simulink model "test_11111"  (R2015a)
settings: Solver=ode45  StartTime=0.0  StopTime=311700  RelTol=1e-3
InitFcn:
  | %% DSPBuilder Start
  | alt_dspbuilder_update_model(bdroot)
  | %% DSPBuilder End
libraries: allblocks_alteradspbuilder2 x104
(part 1 of 2)
settings Model: Creator=ASUS  LastModifiedBy=ASUS

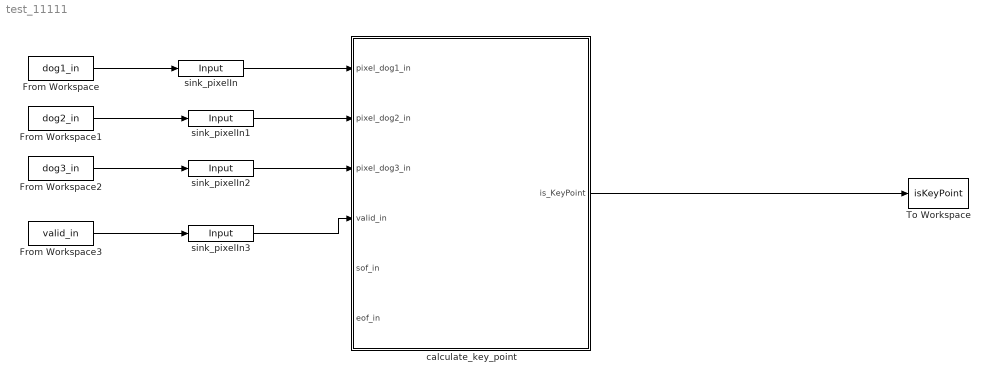
== system test_11111 ==
  From Workspace : FromWorkspace  VariableName=dog1_in  SampleTime=0
  From Workspace1 : FromWorkspace  VariableName=dog2_in  SampleTime=0
  From Workspace2 : FromWorkspace  VariableName=dog3_in  SampleTime=0
  From Workspace3 : FromWorkspace  VariableName=valid_in  SampleTime=0
  To Workspace : ToWorkspace  VariableName=isKeyPoint  SaveFormat=Timeseries  SampleTime=-1
  calculate_key_point : Subsystem
  sink_pixelIn : allblocks_alteradspbuilder2/Input  iofile=C:\Users\ASUS\Desktop\sift_fpga_final\Gaussian filter 5x5\tb_test_11111\test%5F11111_sink%5FpixelIn.salt  BusType=Signed Fractional  bwl=9  bwr=16  SpecifyClock=off  PORTTYPE=Input  externalType=Inferred  allowFloatingPointOverride=on  logOutputs=off
  sink_pixelIn1 : allblocks_alteradspbuilder2/Input  iofile=C:\Users\ASUS\Desktop\sift_fpga_final\Gaussian filter 5x5\tb_test_11111\test%5F11111_sink%5FpixelIn1.salt  BusType=Signed Fractional  bwl=9  bwr=16  SpecifyClock=off  PORTTYPE=Input  externalType=Inferred  allowFloatingPointOverride=on  logOutputs=off
  sink_pixelIn2 : allblocks_alteradspbuilder2/Input  iofile=C:\Users\ASUS\Desktop\sift_fpga_final\Gaussian filter 5x5\tb_test_11111\test%5F11111_sink%5FpixelIn2.salt  BusType=Signed Fractional  bwl=9  bwr=16  SpecifyClock=off  PORTTYPE=Input  externalType=Inferred  allowFloatingPointOverride=on  logOutputs=off
  sink_pixelIn3 : allblocks_alteradspbuilder2/Input  iofile=C:\Users\ASUS\Desktop\sift_fpga_final\Gaussian filter 5x5\tb_test_11111\test%5F11111_sink%5FpixelIn3.salt  BusType=Single Bit  bwl=8  bwr=0  SpecifyClock=off  PORTTYPE=Input  externalType=Inferred  allowFloatingPointOverride=on  logOutputs=off
  wires:
  From Workspace/1 -> sink_pixelIn/1
  From Workspace1/1 -> sink_pixelIn1/1
  From Workspace2/1 -> sink_pixelIn2/1
  From Workspace3/1 -> sink_pixelIn3/1
  calculate_key_point/1(is_KeyPoint) -> To Workspace/1
  sink_pixelIn/1 -> calculate_key_point/1(pixel_dog1_in)
  sink_pixelIn1/1 -> calculate_key_point/2(pixel_dog2_in)
  sink_pixelIn2/1 -> calculate_key_point/3(pixel_dog3_in)
  sink_pixelIn3/1 -> calculate_key_point/4(valid_in)

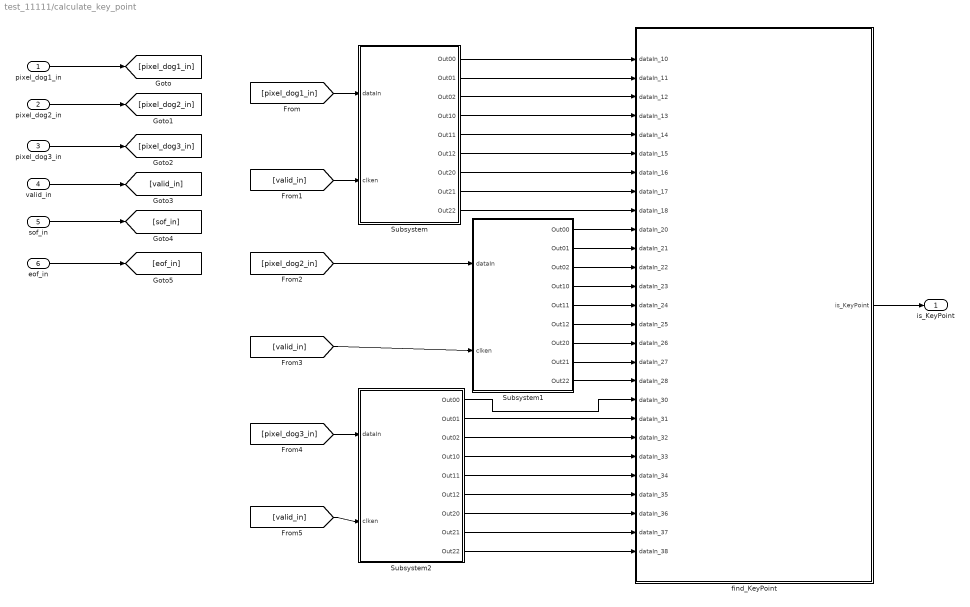
== system test_11111/calculate_key_point ==
  pixel_dog1_in : Inport
  pixel_dog2_in : Inport  Port=2
  pixel_dog3_in : Inport  Port=3
  valid_in : Inport  Port=4
  sof_in : Inport  Port=5
  eof_in : Inport  Port=6
  Subsystem : Subsystem
  Subsystem1 : Subsystem
  Subsystem2 : Subsystem
  find_KeyPoint : Subsystem
  is_KeyPoint : Outport
  wires:
  Subsystem/3(Out02) -> find_KeyPoint/3(dataIn_12)
  Subsystem/6(Out12) -> find_KeyPoint/6(dataIn_15)
  Subsystem/4(Out10) -> find_KeyPoint/4(dataIn_13)
  Subsystem/5(Out11) -> find_KeyPoint/5(dataIn_14)
  Subsystem1/2(Out01) -> find_KeyPoint/11(dataIn_21)
  Subsystem1/3(Out02) -> find_KeyPoint/12(dataIn_22)
  Subsystem1/4(Out10) -> find_KeyPoint/13(dataIn_23)
  Subsystem/2(Out01) -> find_KeyPoint/2(dataIn_11)
  Subsystem2/8(Out21) -> find_KeyPoint/26(dataIn_37)
  Subsystem/8(Out21) -> find_KeyPoint/8(dataIn_17)
  Subsystem/1(Out00) -> find_KeyPoint/1(dataIn_10)
  Subsystem/7(Out20) -> find_KeyPoint/7(dataIn_16)
  Subsystem/9(Out22) -> find_KeyPoint/9(dataIn_18)
  Subsystem1/1(Out00) -> find_KeyPoint/10(dataIn_20)
  find_KeyPoint/1(is_KeyPoint) -> is_KeyPoint/1
  Subsystem2/7(Out20) -> find_KeyPoint/25(dataIn_36)
  [pixel_dog2_in] -> Subsystem1/1(dataIn)
  [pixel_dog1_in] -> Subsystem/1(dataIn)
  eof_in/1 -> [eof_in]
  [valid_in] -> Subsystem2/2(clken)
  valid_in/1 -> [valid_in]
  [valid_in] -> Subsystem1/2(clken)
  pixel_dog2_in/1 -> [pixel_dog2_in]
  pixel_dog1_in/1 -> [pixel_dog1_in]
  sof_in/1 -> [sof_in]
  pixel_dog3_in/1 -> [pixel_dog3_in]
  [valid_in] -> Subsystem/2(clken)
  [pixel_dog3_in] -> Subsystem2/1(dataIn)
  Subsystem2/2(Out01) -> find_KeyPoint/20(dataIn_31)
  Subsystem2/3(Out02) -> find_KeyPoint/21(dataIn_32)
  Subsystem2/4(Out10) -> find_KeyPoint/22(dataIn_33)
  Subsystem2/5(Out11) -> find_KeyPoint/23(dataIn_34)
  Subsystem2/1(Out00) -> find_KeyPoint/19(dataIn_30)
  Subsystem1/5(Out11) -> find_KeyPoint/14(dataIn_24)
  Subsystem1/6(Out12) -> find_KeyPoint/15(dataIn_25)
  Subsystem1/7(Out20) -> find_KeyPoint/16(dataIn_26)
  Subsystem1/8(Out21) -> find_KeyPoint/17(dataIn_27)
  Subsystem2/6(Out12) -> find_KeyPoint/24(dataIn_35)
  Subsystem2/9(Out22) -> find_KeyPoint/27(dataIn_38)
  Subsystem1/9(Out22) -> find_KeyPoint/18(dataIn_28)

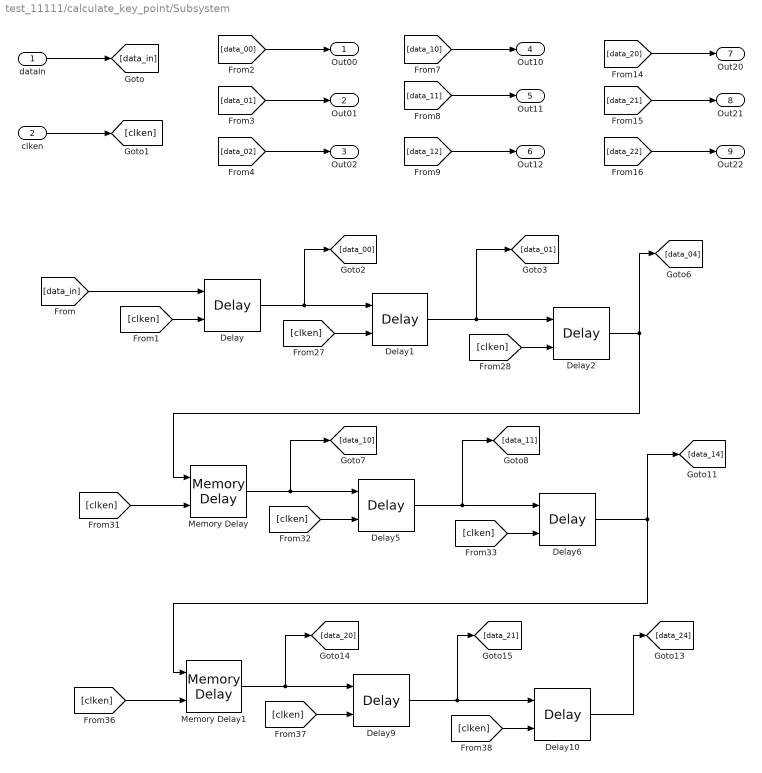
== system test_11111/calculate_key_point/Subsystem ==
  dataIn : Inport
  clken : Inport  Port=2
  Delay : allblocks_alteradspbuilder2/Delay  pipeline=1  pipeline_display=1  ClockPhase=1  use_ena=on  use_sclr=off  allowFloatingPointOverride=on  logOutputs=off  logFile=C:\Users\ASUS\Desktop\sift_fpga_final\Gaussian filter 5x5\tb_test_11111\test%5F11111_calculate%5Fkey%5Fpoint_Subsystem_Delay.fixedpointlog  use_init=off  reset_value=1
  Delay1 : allblocks_alteradspbuilder2/Delay  pipeline=1  pipeline_display=1  ClockPhase=1  use_ena=on  use_sclr=off  allowFloatingPointOverride=on  logOutputs=off  logFile=C:\Users\ASUS\Desktop\sift_fpga_final\Gaussian filter 5x5\tb_test_11111\test%5F11111_calculate%5Fkey%5Fpoint_Subsystem_Delay1.fixedpointlog  use_init=off  reset_value=1
  Delay10 : allblocks_alteradspbuilder2/Delay  pipeline=1  pipeline_display=1  ClockPhase=1  use_ena=on  use_sclr=off  allowFloatingPointOverride=on  logOutputs=off  logFile=C:\Users\ASUS\Desktop\sift_fpga_final\Gaussian filter 5x5\tb_test_11111\test%5F11111_calculate%5Fkey%5Fpoint_Subsystem_Delay10.fixedpointlog  use_init=off  reset_value=1
  Delay2 : allblocks_alteradspbuilder2/Delay  pipeline=1  pipeline_display=1  ClockPhase=1  use_ena=on  use_sclr=off  allowFloatingPointOverride=on  logOutputs=off  logFile=C:\Users\ASUS\Desktop\sift_fpga_final\Gaussian filter 5x5\tb_test_11111\test%5F11111_calculate%5Fkey%5Fpoint_Subsystem_Delay2.fixedpointlog  use_init=off  reset_value=1
  Delay5 : allblocks_alteradspbuilder2/Delay  pipeline=1  pipeline_display=1  ClockPhase=1  use_ena=on  use_sclr=off  allowFloatingPointOverride=on  logOutputs=off  logFile=C:\Users\ASUS\Desktop\sift_fpga_final\Gaussian filter 5x5\tb_test_11111\test%5F11111_calculate%5Fkey%5Fpoint_Subsystem_Delay5.fixedpointlog  use_init=off  reset_value=1
  Delay6 : allblocks_alteradspbuilder2/Delay  pipeline=1  pipeline_display=1  ClockPhase=1  use_ena=on  use_sclr=off  allowFloatingPointOverride=on  logOutputs=off  logFile=C:\Users\ASUS\Desktop\sift_fpga_final\Gaussian filter 5x5\tb_test_11111\test%5F11111_calculate%5Fkey%5Fpoint_Subsystem_Delay6.fixedpointlog  use_init=off  reset_value=1
  Delay9 : allblocks_alteradspbuilder2/Delay  pipeline=1  pipeline_display=1  ClockPhase=1  use_ena=on  use_sclr=off  allowFloatingPointOverride=on  logOutputs=off  logFile=C:\Users\ASUS\Desktop\sift_fpga_final\Gaussian filter 5x5\tb_test_11111\test%5F11111_calculate%5Fkey%5Fpoint_Subsystem_Delay9.fixedpointlog  use_init=off  reset_value=1
  Memory Delay : allblocks_alteradspbuilder2/Memory Delay  BusType=Unsigned Integer  bwl=8  bwr=0  pipeline=638  pipeline_display=638  ram_type=AUTO  use_ena=on  use_sclr=off  allowFloatingPointOverride=on  logOutputs=off  logFile=C:\Users\ASUS\Desktop\sift_fpga_final\Gaussian filter 5x5\tb_test_11111\test%5F11111_calculate%5Fkey%5Fpoint_Subsystem_Memory+Delay.fixedpointlog
  Memory Delay1 : allblocks_alteradspbuilder2/Memory Delay  BusType=Unsigned Integer  bwl=8  bwr=0  pipeline=638  pipeline_display=638  ram_type=AUTO  use_ena=on  use_sclr=off  allowFloatingPointOverride=on  logOutputs=off  logFile=C:\Users\ASUS\Desktop\sift_fpga_final\Gaussian filter 5x5\tb_test_11111\test%5F11111_calculate%5Fkey%5Fpoint_Subsystem_Memory+Delay1.fixedpointlog
  Out00 : Outport
  Out01 : Outport  Port=2
  Out02 : Outport  Port=3
  Out10 : Outport  Port=4
  Out11 : Outport  Port=5
  Out12 : Outport  Port=6
  Out20 : Outport  Port=7
  Out21 : Outport  Port=8
  Out22 : Outport  Port=9
  wires:
  Delay1/1 -> [data_01], Delay2/1
  Delay/1 -> [data_00], Delay1/1
  Delay9/1 -> [data_21], Delay10/1
  [clken] -> Delay10/2
  [clken] -> Memory Delay1/2
  Delay6/1 -> Memory Delay1/1, [data_14]
  Memory Delay1/1 -> [data_20], Delay9/1
  [clken] -> Delay9/2
  [data_02] -> Out02/1
  [clken] -> Delay1/2
  [clken] -> Delay/2
  [data_in] -> Delay/1
  [clken] -> Delay2/2
  Delay2/1 -> Memory Delay/1, [data_04]
  [data_22] -> Out22/1
  Delay10/1 -> [data_24]
  clken/1 -> [clken]
  [data_21] -> Out21/1
  [data_20] -> Out20/1
  [data_10] -> Out10/1
  Memory Delay/1 -> [data_10], Delay5/1
  [clken] -> Memory Delay/2
  [clken] -> Delay6/2
  Delay5/1 -> [data_11], Delay6/1
  [data_12] -> Out12/1
  [data_00] -> Out00/1
  [data_01] -> Out01/1
  [clken] -> Delay5/2
  [data_11] -> Out11/1
  dataIn/1 -> [data_in]

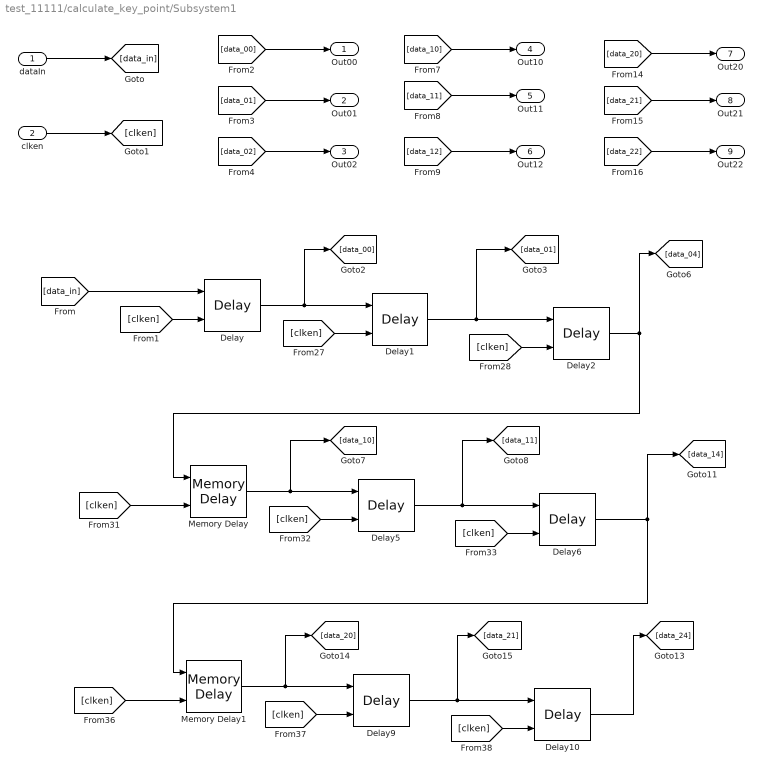
== system test_11111/calculate_key_point/Subsystem1 ==
  dataIn : Inport
  clken : Inport  Port=2
  Delay : allblocks_alteradspbuilder2/Delay  pipeline=1  pipeline_display=1  ClockPhase=1  use_ena=on  use_sclr=off  allowFloatingPointOverride=on  logOutputs=off  logFile=C:\Users\ASUS\Desktop\sift_fpga_final\Gaussian filter 5x5\tb_test_11111\test%5F11111_calculate%5Fkey%5Fpoint_Subsystem1_Delay.fixedpointlog  use_init=off  reset_value=1
  Delay1 : allblocks_alteradspbuilder2/Delay  pipeline=1  pipeline_display=1  ClockPhase=1  use_ena=on  use_sclr=off  allowFloatingPointOverride=on  logOutputs=off  logFile=C:\Users\ASUS\Desktop\sift_fpga_final\Gaussian filter 5x5\tb_test_11111\test%5F11111_calculate%5Fkey%5Fpoint_Subsystem1_Delay1.fixedpointlog  use_init=off  reset_value=1
  Delay10 : allblocks_alteradspbuilder2/Delay  pipeline=1  pipeline_display=1  ClockPhase=1  use_ena=on  use_sclr=off  allowFloatingPointOverride=on  logOutputs=off  logFile=C:\Users\ASUS\Desktop\sift_fpga_final\Gaussian filter 5x5\tb_test_11111\test%5F11111_calculate%5Fkey%5Fpoint_Subsystem1_Delay10.fixedpointlog  use_init=off  reset_value=1
  Delay2 : allblocks_alteradspbuilder2/Delay  pipeline=1  pipeline_display=1  ClockPhase=1  use_ena=on  use_sclr=off  allowFloatingPointOverride=on  logOutputs=off  logFile=C:\Users\ASUS\Desktop\sift_fpga_final\Gaussian filter 5x5\tb_test_11111\test%5F11111_calculate%5Fkey%5Fpoint_Subsystem1_Delay2.fixedpointlog  use_init=off  reset_value=1
  Delay5 : allblocks_alteradspbuilder2/Delay  pipeline=1  pipeline_display=1  ClockPhase=1  use_ena=on  use_sclr=off  allowFloatingPointOverride=on  logOutputs=off  logFile=C:\Users\ASUS\Desktop\sift_fpga_final\Gaussian filter 5x5\tb_test_11111\test%5F11111_calculate%5Fkey%5Fpoint_Subsystem1_Delay5.fixedpointlog  use_init=off  reset_value=1
  Delay6 : allblocks_alteradspbuilder2/Delay  pipeline=1  pipeline_display=1  ClockPhase=1  use_ena=on  use_sclr=off  allowFloatingPointOverride=on  logOutputs=off  logFile=C:\Users\ASUS\Desktop\sift_fpga_final\Gaussian filter 5x5\tb_test_11111\test%5F11111_calculate%5Fkey%5Fpoint_Subsystem1_Delay6.fixedpointlog  use_init=off  reset_value=1
  Delay9 : allblocks_alteradspbuilder2/Delay  pipeline=1  pipeline_display=1  ClockPhase=1  use_ena=on  use_sclr=off  allowFloatingPointOverride=on  logOutputs=off  logFile=C:\Users\ASUS\Desktop\sift_fpga_final\Gaussian filter 5x5\tb_test_11111\test%5F11111_calculate%5Fkey%5Fpoint_Subsystem1_Delay9.fixedpointlog  use_init=off  reset_value=1
  Memory Delay : allblocks_alteradspbuilder2/Memory Delay  BusType=Unsigned Integer  bwl=8  bwr=0  pipeline=638  pipeline_display=638  ram_type=AUTO  use_ena=on  use_sclr=off  allowFloatingPointOverride=on  logOutputs=off  logFile=C:\Users\ASUS\Desktop\sift_fpga_final\Gaussian filter 5x5\tb_test_11111\test%5F11111_calculate%5Fkey%5Fpoint_Subsystem1_Memory+Delay.fixedpointlog
  Memory Delay1 : allblocks_alteradspbuilder2/Memory Delay  BusType=Unsigned Integer  bwl=8  bwr=0  pipeline=638  pipeline_display=638  ram_type=AUTO  use_ena=on  use_sclr=off  allowFloatingPointOverride=on  logOutputs=off  logFile=C:\Users\ASUS\Desktop\sift_fpga_final\Gaussian filter 5x5\tb_test_11111\test%5F11111_calculate%5Fkey%5Fpoint_Subsystem1_Memory+Delay1.fixedpointlog
  Out00 : Outport
  Out01 : Outport  Port=2
  Out02 : Outport  Port=3
  Out10 : Outport  Port=4
  Out11 : Outport  Port=5
  Out12 : Outport  Port=6
  Out20 : Outport  Port=7
  Out21 : Outport  Port=8
  Out22 : Outport  Port=9
  wires:
  Delay1/1 -> [data_01], Delay2/1
  Delay/1 -> [data_00], Delay1/1
  Delay9/1 -> [data_21], Delay10/1
  [clken] -> Delay10/2
  [clken] -> Memory Delay1/2
  Delay6/1 -> Memory Delay1/1, [data_14]
  Memory Delay1/1 -> [data_20], Delay9/1
  [clken] -> Delay9/2
  [data_02] -> Out02/1
  [clken] -> Delay1/2
  [clken] -> Delay/2
  [data_in] -> Delay/1
  [clken] -> Delay2/2
  Delay2/1 -> Memory Delay/1, [data_04]
  [data_22] -> Out22/1
  Delay10/1 -> [data_24]
  clken/1 -> [clken]
  [data_21] -> Out21/1
  [data_20] -> Out20/1
  [data_10] -> Out10/1
  Memory Delay/1 -> [data_10], Delay5/1
  [clken] -> Memory Delay/2
  [clken] -> Delay6/2
  Delay5/1 -> [data_11], Delay6/1
  [data_12] -> Out12/1
  [data_00] -> Out00/1
  [data_01] -> Out01/1
  [clken] -> Delay5/2
  [data_11] -> Out11/1
  dataIn/1 -> [data_in]

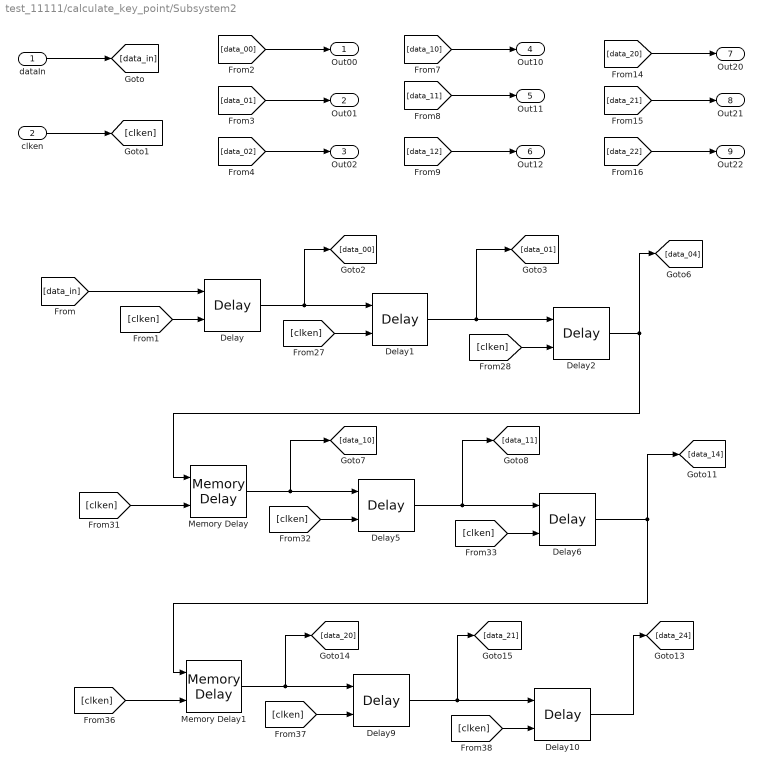
== system test_11111/calculate_key_point/Subsystem2 ==
  dataIn : Inport
  clken : Inport  Port=2
  Delay : allblocks_alteradspbuilder2/Delay  pipeline=1  pipeline_display=1  ClockPhase=1  use_ena=on  use_sclr=off  allowFloatingPointOverride=on  logOutputs=off  logFile=C:\Users\ASUS\Desktop\sift_fpga_final\Gaussian filter 5x5\tb_test_11111\test%5F11111_calculate%5Fkey%5Fpoint_Subsystem2_Delay.fixedpointlog  use_init=off  reset_value=1
  Delay1 : allblocks_alteradspbuilder2/Delay  pipeline=1  pipeline_display=1  ClockPhase=1  use_ena=on  use_sclr=off  allowFloatingPointOverride=on  logOutputs=off  logFile=C:\Users\ASUS\Desktop\sift_fpga_final\Gaussian filter 5x5\tb_test_11111\test%5F11111_calculate%5Fkey%5Fpoint_Subsystem2_Delay1.fixedpointlog  use_init=off  reset_value=1
  Delay10 : allblocks_alteradspbuilder2/Delay  pipeline=1  pipeline_display=1  ClockPhase=1  use_ena=on  use_sclr=off  allowFloatingPointOverride=on  logOutputs=off  logFile=C:\Users\ASUS\Desktop\sift_fpga_final\Gaussian filter 5x5\tb_test_11111\test%5F11111_calculate%5Fkey%5Fpoint_Subsystem2_Delay10.fixedpointlog  use_init=off  reset_value=1
  Delay2 : allblocks_alteradspbuilder2/Delay  pipeline=1  pipeline_display=1  ClockPhase=1  use_ena=on  use_sclr=off  allowFloatingPointOverride=on  logOutputs=off  logFile=C:\Users\ASUS\Desktop\sift_fpga_final\Gaussian filter 5x5\tb_test_11111\test%5F11111_calculate%5Fkey%5Fpoint_Subsystem2_Delay2.fixedpointlog  use_init=off  reset_value=1
  Delay5 : allblocks_alteradspbuilder2/Delay  pipeline=1  pipeline_display=1  ClockPhase=1  use_ena=on  use_sclr=off  allowFloatingPointOverride=on  logOutputs=off  logFile=C:\Users\ASUS\Desktop\sift_fpga_final\Gaussian filter 5x5\tb_test_11111\test%5F11111_calculate%5Fkey%5Fpoint_Subsystem2_Delay5.fixedpointlog  use_init=off  reset_value=1
  Delay6 : allblocks_alteradspbuilder2/Delay  pipeline=1  pipeline_display=1  ClockPhase=1  use_ena=on  use_sclr=off  allowFloatingPointOverride=on  logOutputs=off  logFile=C:\Users\ASUS\Desktop\sift_fpga_final\Gaussian filter 5x5\tb_test_11111\test%5F11111_calculate%5Fkey%5Fpoint_Subsystem2_Delay6.fixedpointlog  use_init=off  reset_value=1
  Delay9 : allblocks_alteradspbuilder2/Delay  pipeline=1  pipeline_display=1  ClockPhase=1  use_ena=on  use_sclr=off  allowFloatingPointOverride=on  logOutputs=off  logFile=C:\Users\ASUS\Desktop\sift_fpga_final\Gaussian filter 5x5\tb_test_11111\test%5F11111_calculate%5Fkey%5Fpoint_Subsystem2_Delay9.fixedpointlog  use_init=off  reset_value=1
  Memory Delay : allblocks_alteradspbuilder2/Memory Delay  BusType=Unsigned Integer  bwl=8  bwr=0  pipeline=638  pipeline_display=638  ram_type=AUTO  use_ena=on  use_sclr=off  allowFloatingPointOverride=on  logOutputs=off  logFile=C:\Users\ASUS\Desktop\sift_fpga_final\Gaussian filter 5x5\tb_test_11111\test%5F11111_calculate%5Fkey%5Fpoint_Subsystem2_Memory+Delay.fixedpointlog
  Memory Delay1 : allblocks_alteradspbuilder2/Memory Delay  BusType=Unsigned Integer  bwl=8  bwr=0  pipeline=638  pipeline_display=638  ram_type=AUTO  use_ena=on  use_sclr=off  allowFloatingPointOverride=on  logOutputs=off  logFile=C:\Users\ASUS\Desktop\sift_fpga_final\Gaussian filter 5x5\tb_test_11111\test%5F11111_calculate%5Fkey%5Fpoint_Subsystem2_Memory+Delay1.fixedpointlog
  Out00 : Outport
  Out01 : Outport  Port=2
  Out02 : Outport  Port=3
  Out10 : Outport  Port=4
  Out11 : Outport  Port=5
  Out12 : Outport  Port=6
  Out20 : Outport  Port=7
  Out21 : Outport  Port=8
  Out22 : Outport  Port=9
  wires:
  Delay1/1 -> [data_01], Delay2/1
  Delay/1 -> [data_00], Delay1/1
  Delay9/1 -> [data_21], Delay10/1
  [clken] -> Delay10/2
  [clken] -> Memory Delay1/2
  Delay6/1 -> Memory Delay1/1, [data_14]
  Memory Delay1/1 -> [data_20], Delay9/1
  [clken] -> Delay9/2
  [data_02] -> Out02/1
  [clken] -> Delay1/2
  [clken] -> Delay/2
  [data_in] -> Delay/1
  [clken] -> Delay2/2
  Delay2/1 -> Memory Delay/1, [data_04]
  [data_22] -> Out22/1
  Delay10/1 -> [data_24]
  clken/1 -> [clken]
  [data_21] -> Out21/1
  [data_20] -> Out20/1
  [data_10] -> Out10/1
  Memory Delay/1 -> [data_10], Delay5/1
  [clken] -> Memory Delay/2
  [clken] -> Delay6/2
  Delay5/1 -> [data_11], Delay6/1
  [data_12] -> Out12/1
  [data_00] -> Out00/1
  [data_01] -> Out01/1
  [clken] -> Delay5/2
  [data_11] -> Out11/1
  dataIn/1 -> [data_in]

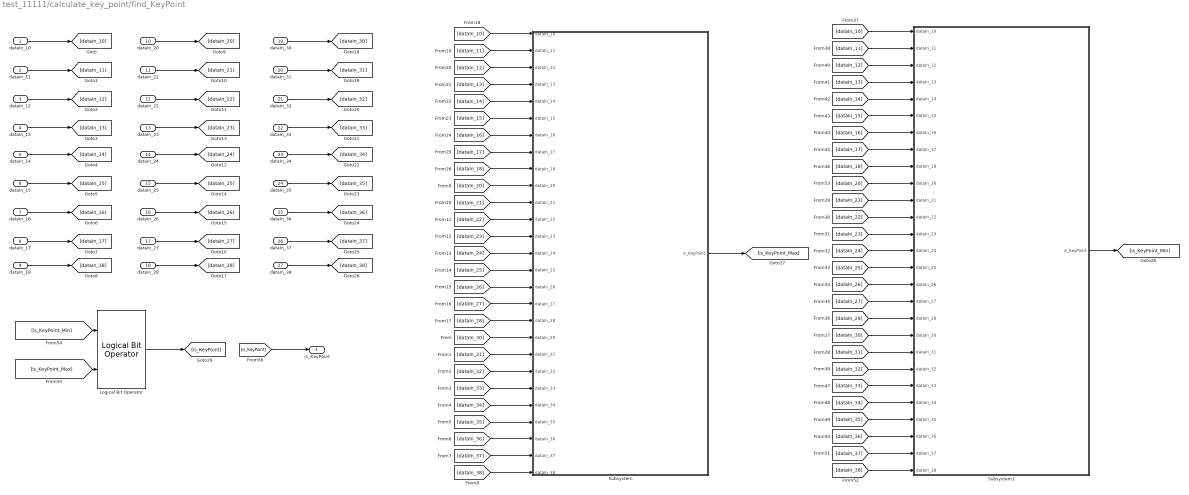
== system test_11111/calculate_key_point/find_KeyPoint ==
  dataIn_10 : Inport
  dataIn_11 : Inport  Port=2
  dataIn_12 : Inport  Port=3
  dataIn_13 : Inport  Port=4
  dataIn_14 : Inport  Port=5
  dataIn_15 : Inport  Port=6
  dataIn_16 : Inport  Port=7
  dataIn_17 : Inport  Port=8
  dataIn_18 : Inport  Port=9
  dataIn_20 : Inport  Port=10
  dataIn_21 : Inport  Port=11
  dataIn_22 : Inport  Port=12
  dataIn_23 : Inport  Port=13
  dataIn_24 : Inport  Port=14
  dataIn_25 : Inport  Port=15
  dataIn_26 : Inport  Port=16
  dataIn_27 : Inport  Port=17
  dataIn_28 : Inport  Port=18
  dataIn_30 : Inport  Port=19
  dataIn_31 : Inport  Port=20
  dataIn_32 : Inport  Port=21
  dataIn_33 : Inport  Port=22
  dataIn_34 : Inport  Port=23
  dataIn_35 : Inport  Port=24
  dataIn_36 : Inport  Port=25
  dataIn_37 : Inport  Port=26
  dataIn_38 : Inport  Port=27
  Logical Bit Operator : allblocks_alteradspbuilder2/Logical Bit Operator  LogicalOperator=OR  user_inputs=2  pipeline_display=0
  Subsystem : Subsystem
  Subsystem1 : Subsystem
  is_KeyPoint : Outport
  wires:
  [dataIn_32] -> Subsystem/21(dataIn_32)
  [dataIn_33] -> Subsystem/22(dataIn_33)
  [dataIn_36] -> Subsystem/25(dataIn_36)
  [dataIn_37] -> Subsystem/26(dataIn_37)
  [dataIn_34] -> Subsystem/23(dataIn_34)
  [dataIn_35] -> Subsystem/24(dataIn_35)
  [dataIn_30] -> Subsystem/19(dataIn_30)
  [dataIn_31] -> Subsystem/20(dataIn_31)
  [is_KeyPoint_Max] -> Logical Bit Operator/2
  [is_KeyPoint_Min] -> Logical Bit Operator/1
  Subsystem/1(is_KeyPoint) -> [is_KeyPoint_Max]
  [dataIn_28] -> Subsystem/18(dataIn_28)
  [dataIn_26] -> Subsystem/16(dataIn_26)
  [dataIn_22] -> Subsystem/12(dataIn_22)
  [dataIn_27] -> Subsystem/17(dataIn_27)
  [dataIn_20] -> Subsystem/10(dataIn_20)
  [dataIn_23] -> Subsystem/13(dataIn_23)
  [dataIn_24] -> Subsystem/14(dataIn_24)
  [dataIn_21] -> Subsystem/11(dataIn_21)
  [dataIn_25] -> Subsystem/15(dataIn_25)
  [dataIn_10] -> Subsystem/1(dataIn_10)
  [dataIn_11] -> Subsystem/2(dataIn_11)
  [dataIn_12] -> Subsystem/3(dataIn_12)
  dataIn_23/1 -> [dataIn_23]
  dataIn_17/1 -> [dataIn_17]
  dataIn_22/1 -> [dataIn_22]
  dataIn_14/1 -> [dataIn_14]
  dataIn_16/1 -> [dataIn_16]
  dataIn_28/1 -> [dataIn_28]
  dataIn_20/1 -> [dataIn_20]
  dataIn_21/1 -> [dataIn_21]
  dataIn_26/1 -> [dataIn_26]
  dataIn_10/1 -> [dataIn_10]
  dataIn_30/1 -> [dataIn_30]
  dataIn_27/1 -> [dataIn_27]
  dataIn_25/1 -> [dataIn_25]
  dataIn_15/1 -> [dataIn_15]
  dataIn_18/1 -> [dataIn_18]
  dataIn_24/1 -> [dataIn_24]
  dataIn_32/1 -> [dataIn_32]
  dataIn_13/1 -> [dataIn_13]
  dataIn_31/1 -> [dataIn_31]
  [dataIn_14] -> Subsystem/5(dataIn_14)
  dataIn_34/1 -> [dataIn_34]
  dataIn_11/1 -> [dataIn_11]
  [dataIn_17] -> Subsystem/8(dataIn_17)
  dataIn_35/1 -> [dataIn_35]
  dataIn_33/1 -> [dataIn_33]
  dataIn_38/1 -> [dataIn_38]
  [dataIn_13] -> Subsystem/4(dataIn_13)
  [dataIn_16] -> Subsystem/7(dataIn_16)
  [dataIn_15] -> Subsystem/6(dataIn_15)
  dataIn_12/1 -> [dataIn_12]
  [dataIn_18] -> Subsystem/9(dataIn_18)
  dataIn_36/1 -> [dataIn_36]
  dataIn_37/1 -> [dataIn_37]
  [dataIn_38] -> Subsystem/27(dataIn_38)
  Subsystem1/1(is_KeyPoint) -> [is_KeyPoint_Min]
  [dataIn_11] -> Subsystem1/2(dataIn_11)
  [dataIn_12] -> Subsystem1/3(dataIn_12)
  [dataIn_13] -> Subsystem1/4(dataIn_13)
  [dataIn_15] -> Subsystem1/6(dataIn_15)
  [dataIn_16] -> Subsystem1/7(dataIn_16)
  [dataIn_17] -> Subsystem1/8(dataIn_17)
  [dataIn_18] -> Subsystem1/9(dataIn_18)
  [dataIn_31] -> Subsystem1/20(dataIn_31)
  [dataIn_14] -> Subsystem1/5(dataIn_14)
  [is_KeyPoint] -> is_KeyPoint/1
  [dataIn_33] -> Subsystem1/22(dataIn_33)
  [dataIn_32] -> Subsystem1/21(dataIn_32)
  [dataIn_34] -> Subsystem1/23(dataIn_34)
  [dataIn_35] -> Subsystem1/24(dataIn_35)
  [dataIn_36] -> Subsystem1/25(dataIn_36)
  [dataIn_21] -> Subsystem1/11(dataIn_21)
  [dataIn_22] -> Subsystem1/12(dataIn_22)
  [dataIn_23] -> Subsystem1/13(dataIn_23)
  [dataIn_25] -> Subsystem1/15(dataIn_25)
  [dataIn_24] -> Subsystem1/14(dataIn_24)
  [dataIn_38] -> Subsystem1/27(dataIn_38)
  [dataIn_20] -> Subsystem1/10(dataIn_20)
  [dataIn_26] -> Subsystem1/16(dataIn_26)
  [dataIn_30] -> Subsystem1/19(dataIn_30)
  [dataIn_27] -> Subsystem1/17(dataIn_27)
  [dataIn_37] -> Subsystem1/26(dataIn_37)
  [dataIn_28] -> Subsystem1/18(dataIn_28)
  [dataIn_10] -> Subsystem1/1(dataIn_10)
  Logical Bit Operator/1 -> [is_KeyPoint]

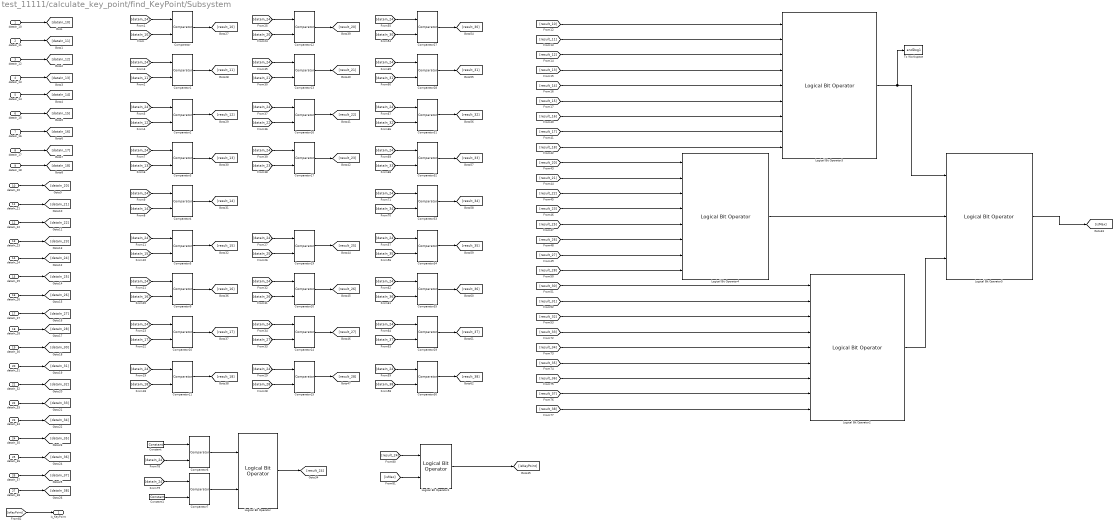
== system test_11111/calculate_key_point/find_KeyPoint/Subsystem ==
  dataIn_10 : Inport
  dataIn_11 : Inport  Port=2
  dataIn_12 : Inport  Port=3
  dataIn_13 : Inport  Port=4
  dataIn_14 : Inport  Port=5
  dataIn_15 : Inport  Port=6
  dataIn_16 : Inport  Port=7
  dataIn_17 : Inport  Port=8
  dataIn_18 : Inport  Port=9
  dataIn_20 : Inport  Port=10
  dataIn_21 : Inport  Port=11
  dataIn_22 : Inport  Port=12
  dataIn_23 : Inport  Port=13
  dataIn_24 : Inport  Port=14
  dataIn_25 : Inport  Port=15
  dataIn_26 : Inport  Port=16
  dataIn_27 : Inport  Port=17
  dataIn_28 : Inport  Port=18
  dataIn_30 : Inport  Port=19
  dataIn_31 : Inport  Port=20
  dataIn_32 : Inport  Port=21
  dataIn_33 : Inport  Port=22
  dataIn_34 : Inport  Port=23
  dataIn_35 : Inport  Port=24
  dataIn_36 : Inport  Port=25
  dataIn_37 : Inport  Port=26
  dataIn_38 : Inport  Port=27
  Comparator : allblocks_alteradspbuilder2/Comparator  direction=a > b  pipeline_display=0  allowFloatingPointOverride=on  logOutputs=off  logFile=C:\Users\ASUS\Desktop\sift_fpga_final\Gaussian filter 5x5\tb_test_11111\test%5F11111_calculate%5Fkey%5Fpoint_find%5FKeyPoint_Subsystem_Comparator.fixedpointlog
  Comparator1 : allblocks_alteradspbuilder2/Comparator  direction=a > b  pipeline_display=0  allowFloatingPointOverride=on  logOutputs=off  logFile=C:\Users\ASUS\Desktop\sift_fpga_final\Gaussian filter 5x5\tb_test_11111\test%5F11111_calculate%5Fkey%5Fpoint_find%5FKeyPoint_Subsystem_Comparator1.fixedpointlog
  Comparator10 : allblocks_alteradspbuilder2/Comparator  direction=a > b  pipeline_display=0  allowFloatingPointOverride=on  logOutputs=off  logFile=C:\Users\ASUS\Desktop\sift_fpga_final\Gaussian filter 5x5\tb_test_11111\test%5F11111_calculate%5Fkey%5Fpoint_find%5FKeyPoint_Subsystem_Comparator10.fixedpointlog
  Comparator11 : allblocks_alteradspbuilder2/Comparator  direction=a > b  pipeline_display=0  allowFloatingPointOverride=on  logOutputs=off  logFile=C:\Users\ASUS\Desktop\sift_fpga_final\Gaussian filter 5x5\tb_test_11111\test%5F11111_calculate%5Fkey%5Fpoint_find%5FKeyPoint_Subsystem_Comparator11.fixedpointlog
  Comparator12 : allblocks_alteradspbuilder2/Comparator  direction=a > b  pipeline_display=0  allowFloatingPointOverride=on  logOutputs=off  logFile=C:\Users\ASUS\Desktop\sift_fpga_final\Gaussian filter 5x5\tb_test_11111\test%5F11111_calculate%5Fkey%5Fpoint_find%5FKeyPoint_Subsystem_Comparator12.fixedpointlog
  Comparator13 : allblocks_alteradspbuilder2/Comparator  direction=a > b  pipeline_display=0  allowFloatingPointOverride=on  logOutputs=off  logFile=C:\Users\ASUS\Desktop\sift_fpga_final\Gaussian filter 5x5\tb_test_11111\test%5F11111_calculate%5Fkey%5Fpoint_find%5FKeyPoint_Subsystem_Comparator13.fixedpointlog
  Comparator14 : allblocks_alteradspbuilder2/Comparator  direction=a > b  pipeline_display=0  allowFloatingPointOverride=on  logOutputs=off  logFile=C:\Users\ASUS\Desktop\sift_fpga_final\Gaussian filter 5x5\tb_test_11111\test%5F11111_calculate%5Fkey%5Fpoint_find%5FKeyPoint_Subsystem_Comparator14.fixedpointlog
  Comparator15 : allblocks_alteradspbuilder2/Comparator  direction=a > b  pipeline_display=0  allowFloatingPointOverride=on  logOutputs=off  logFile=C:\Users\ASUS\Desktop\sift_fpga_final\Gaussian filter 5x5\tb_test_11111\test%5F11111_calculate%5Fkey%5Fpoint_find%5FKeyPoint_Subsystem_Comparator15.fixedpointlog
  Comparator16 : allblocks_alteradspbuilder2/Comparator  direction=a > b  pipeline_display=0  allowFloatingPointOverride=on  logOutputs=off  logFile=C:\Users\ASUS\Desktop\sift_fpga_final\Gaussian filter 5x5\tb_test_11111\test%5F11111_calculate%5Fkey%5Fpoint_find%5FKeyPoint_Subsystem_Comparator16.fixedpointlog
  Comparator17 : allblocks_alteradspbuilder2/Comparator  direction=a > b  pipeline_display=0  allowFloatingPointOverride=on  logOutputs=off  logFile=C:\Users\ASUS\Desktop\sift_fpga_final\Gaussian filter 5x5\tb_test_11111\test%5F11111_calculate%5Fkey%5Fpoint_find%5FKeyPoint_Subsystem_Comparator17.fixedpointlog
  Comparator19 : allblocks_alteradspbuilder2/Comparator  direction=a > b  pipeline_display=0  allowFloatingPointOverride=on  logOutputs=off  logFile=C:\Users\ASUS\Desktop\sift_fpga_final\Gaussian filter 5x5\tb_test_11111\test%5F11111_calculate%5Fkey%5Fpoint_find%5FKeyPoint_Subsystem_Comparator19.fixedpointlog
  Comparator2 : allblocks_alteradspbuilder2/Comparator  direction=a > b  pipeline_display=0  allowFloatingPointOverride=on  logOutputs=off  logFile=C:\Users\ASUS\Desktop\sift_fpga_final\Gaussian filter 5x5\tb_test_11111\test%5F11111_calculate%5Fkey%5Fpoint_find%5FKeyPoint_Subsystem_Comparator2.fixedpointlog
  Comparator20 : allblocks_alteradspbuilder2/Comparator  direction=a > b  pipeline_display=0  allowFloatingPointOverride=on  logOutputs=off  logFile=C:\Users\ASUS\Desktop\sift_fpga_final\Gaussian filter 5x5\tb_test_11111\test%5F11111_calculate%5Fkey%5Fpoint_find%5FKeyPoint_Subsystem_Comparator20.fixedpointlog
  Comparator27 : allblocks_alteradspbuilder2/Comparator  direction=a > b  pipeline_display=0  allowFloatingPointOverride=on  logOutputs=off  logFile=C:\Users\ASUS\Desktop\sift_fpga_final\Gaussian filter 5x5\tb_test_11111\test%5F11111_calculate%5Fkey%5Fpoint_find%5FKeyPoint_Subsystem_Comparator27.fixedpointlog
  Comparator28 : allblocks_alteradspbuilder2/Comparator  direction=a > b  pipeline_display=0  allowFloatingPointOverride=on  logOutputs=off  logFile=C:\Users\ASUS\Desktop\sift_fpga_final\Gaussian filter 5x5\tb_test_11111\test%5F11111_calculate%5Fkey%5Fpoint_find%5FKeyPoint_Subsystem_Comparator28.fixedpointlog
  Comparator29 : allblocks_alteradspbuilder2/Comparator  direction=a > b  pipeline_display=0  allowFloatingPointOverride=on  logOutputs=off  logFile=C:\Users\ASUS\Desktop\sift_fpga_final\Gaussian filter 5x5\tb_test_11111\test%5F11111_calculate%5Fkey%5Fpoint_find%5FKeyPoint_Subsystem_Comparator29.fixedpointlog
  Comparator3 : allblocks_alteradspbuilder2/Comparator  direction=a > b  pipeline_display=0  allowFloatingPointOverride=on  logOutputs=off  logFile=C:\Users\ASUS\Desktop\sift_fpga_final\Gaussian filter 5x5\tb_test_11111\test%5F11111_calculate%5Fkey%5Fpoint_find%5FKeyPoint_Subsystem_Comparator3.fixedpointlog
  Comparator30 : allblocks_alteradspbuilder2/Comparator  direction=a > b  pipeline_display=0  allowFloatingPointOverride=on  logOutputs=off  logFile=C:\Users\ASUS\Desktop\sift_fpga_final\Gaussian filter 5x5\tb_test_11111\test%5F11111_calculate%5Fkey%5Fpoint_find%5FKeyPoint_Subsystem_Comparator30.fixedpointlog
  Comparator31 : allblocks_alteradspbuilder2/Comparator  direction=a > b  pipeline_display=0  allowFloatingPointOverride=on  logOutputs=off  logFile=C:\Users\ASUS\Desktop\sift_fpga_final\Gaussian filter 5x5\tb_test_11111\test%5F11111_calculate%5Fkey%5Fpoint_find%5FKeyPoint_Subsystem_Comparator31.fixedpointlog
  Comparator32 : allblocks_alteradspbuilder2/Comparator  direction=a > b  pipeline_display=0  allowFloatingPointOverride=on  logOutputs=off  logFile=C:\Users\ASUS\Desktop\sift_fpga_final\Gaussian filter 5x5\tb_test_11111\test%5F11111_calculate%5Fkey%5Fpoint_find%5FKeyPoint_Subsystem_Comparator32.fixedpointlog
  Comparator33 : allblocks_alteradspbuilder2/Comparator  direction=a > b  pipeline_display=0  allowFloatingPointOverride=on  logOutputs=off  logFile=C:\Users\ASUS\Desktop\sift_fpga_final\Gaussian filter 5x5\tb_test_11111\test%5F11111_calculate%5Fkey%5Fpoint_find%5FKeyPoint_Subsystem_Comparator33.fixedpointlog
  Comparator34 : allblocks_alteradspbuilder2/Comparator  direction=a > b  pipeline_display=0  allowFloatingPointOverride=on  logOutputs=off  logFile=C:\Users\ASUS\Desktop\sift_fpga_final\Gaussian filter 5x5\tb_test_11111\test%5F11111_calculate%5Fkey%5Fpoint_find%5FKeyPoint_Subsystem_Comparator34.fixedpointlog
  Comparator35 : allblocks_alteradspbuilder2/Comparator  direction=a > b  pipeline_display=0  allowFloatingPointOverride=on  logOutputs=off  logFile=C:\Users\ASUS\Desktop\sift_fpga_final\Gaussian filter 5x5\tb_test_11111\test%5F11111_calculate%5Fkey%5Fpoint_find%5FKeyPoint_Subsystem_Comparator35.fixedpointlog
  Comparator4 : allblocks_alteradspbuilder2/Comparator  direction=a > b  pipeline_display=0  allowFloatingPointOverride=on  logOutputs=off  logFile=C:\Users\ASUS\Desktop\sift_fpga_final\Gaussian filter 5x5\tb_test_11111\test%5F11111_calculate%5Fkey%5Fpoint_find%5FKeyPoint_Subsystem_Comparator4.fixedpointlog
  Comparator5 : allblocks_alteradspbuilder2/Comparator  direction=a > b  pipeline_display=0  allowFloatingPointOverride=on  logOutputs=off  logFile=C:\Users\ASUS\Desktop\sift_fpga_final\Gaussian filter 5x5\tb_test_11111\test%5F11111_calculate%5Fkey%5Fpoint_find%5FKeyPoint_Subsystem_Comparator5.fixedpointlog
  Comparator6 : allblocks_alteradspbuilder2/Comparator  direction=a > b  pipeline_display=0  allowFloatingPointOverride=on  logOutputs=off  logFile=C:\Users\ASUS\Desktop\sift_fpga_final\Gaussian filter 5x5\tb_test_11111\test%5F11111_calculate%5Fkey%5Fpoint_find%5FKeyPoint_Subsystem_Comparator6.fixedpointlog
  Comparator7 : allblocks_alteradspbuilder2/Comparator  direction=a > b  pipeline_display=0  allowFloatingPointOverride=on  logOutputs=off  logFile=C:\Users\ASUS\Desktop\sift_fpga_final\Gaussian filter 5x5\tb_test_11111\test%5F11111_calculate%5Fkey%5Fpoint_find%5FKeyPoint_Subsystem_Comparator7.fixedpointlog
  Comparator9 : allblocks_alteradspbuilder2/Comparator  direction=a > b  pipeline_display=0  allowFloatingPointOverride=on  logOutputs=off  logFile=C:\Users\ASUS\Desktop\sift_fpga_final\Gaussian filter 5x5\tb_test_11111\test%5F11111_calculate%5Fkey%5Fpoint_find%5FKeyPoint_Subsystem_Comparator9.fixedpointlog
  Constant : allblocks_alteradspbuilder2/Constant  mask_cst=0.8*0.015  BusType=Signed Fractional  bwl=9  bwr=16  roundMode=Truncate  satMode=Wrap  SpecifyClock=off  allowFloatingPointOverride=on  logOutputs=off  logFile=C:\Users\ASUS\Desktop\sift_fpga_final\Gaussian filter 5x5\tb_test_11111\test%5F11111_calculate%5Fkey%5Fpoint_find%5FKeyPoint_Subsystem_Constant.fixedpointlog
  Constant1 : allblocks_alteradspbuilder2/Constant  mask_cst=-0.8*0.015  BusType=Signed Fractional  bwl=9  bwr=16  roundMode=Truncate  satMode=Wrap  SpecifyClock=off  allowFloatingPointOverride=on  logOutputs=off  logFile=C:\Users\ASUS\Desktop\sift_fpga_final\Gaussian filter 5x5\tb_test_11111\test%5F11111_calculate%5Fkey%5Fpoint_find%5FKeyPoint_Subsystem_Constant1.fixedpointlog
  Logical Bit Operator : allblocks_alteradspbuilder2/Logical Bit Operator  LogicalOperator=OR  user_inputs=2  pipeline_display=0
  Logical Bit Operator1 : allblocks_alteradspbuilder2/Logical Bit Operator  LogicalOperator=AND  user_inputs=2  pipeline_display=0
  Logical Bit Operator2 : allblocks_alteradspbuilder2/Logical Bit Operator  LogicalOperator=AND  user_inputs=9  pipeline_display=0
  Logical Bit Operator3 : allblocks_alteradspbuilder2/Logical Bit Operator  LogicalOperator=AND  user_inputs=9  pipeline_display=0
  Logical Bit Operator4 : allblocks_alteradspbuilder2/Logical Bit Operator  LogicalOperator=AND  user_inputs=8  pipeline_display=0
  Logical Bit Operator5 : allblocks_alteradspbuilder2/Logical Bit Operator  LogicalOperator=AND  user_inputs=3  pipeline_display=0
  To Workspace : ToWorkspace  VariableName=andDog1  SaveFormat=Timeseries  SampleTime=-1
  is_KeyPoint : Outport
  wires:
  dataIn_18/1 -> [dataIn_18]
  dataIn_10/1 -> [dataIn_10]
  [result_10] -> Logical Bit Operator3/1
  [dataIn_24] -> Comparator/1
  Comparator1/1 -> [result_11]
  [dataIn_10] -> Comparator/2
  [dataIn_24] -> Comparator1/1
  [dataIn_11] -> Comparator1/2
  [result_20] -> Logical Bit Operator4/1
  [result_28] -> Logical Bit Operator4/8
  [result_30] -> Logical Bit Operator2/1
  [result_31] -> Logical Bit Operator2/2
  [result_33] -> Logical Bit Operator2/4
  [result_34] -> Logical Bit Operator2/5
  [result_36] -> Logical Bit Operator2/7
  [result_35] -> Logical Bit Operator2/6
  [result_32] -> Logical Bit Operator2/3
  [result_37] -> Logical Bit Operator2/8
  [result_11] -> Logical Bit Operator3/2
  [result_38] -> Logical Bit Operator2/9
  [result_22] -> Logical Bit Operator4/3
  [result_26] -> Logical Bit Operator4/6
  [result_23] -> Logical Bit Operator4/4
  Comparator7/1 -> Logical Bit Operator/2
  [isMax] -> Logical Bit Operator1/2
  [dataIn_24] -> Comparator2/1
  [dataIn_24] -> Comparator6/2
  Comparator2/1 -> [result_12]
  [dataIn_12] -> Comparator2/2
  [result_21] -> Logical Bit Operator4/2
  [result_25] -> Logical Bit Operator4/5
  [dataIn_24] -> Comparator9/1
  Comparator9/1 -> [result_16]
  [dataIn_24] -> Comparator10/1
  [dataIn_16] -> Comparator9/2
  Comparator10/1 -> [result_17]
  [dataIn_17] -> Comparator10/2
  [dataIn_24] -> Comparator11/1
  Comparator11/1 -> [result_18]
  [dataIn_18] -> Comparator11/2
  dataIn_14/1 -> [dataIn_14]
  dataIn_15/1 -> [dataIn_15]
  dataIn_17/1 -> [dataIn_17]
  dataIn_16/1 -> [dataIn_16]
  dataIn_24/1 -> [dataIn_24]
  dataIn_27/1 -> [dataIn_27]
  dataIn_28/1 -> [dataIn_28]
  dataIn_25/1 -> [dataIn_25]
  dataIn_22/1 -> [dataIn_22]
  dataIn_20/1 -> [dataIn_20]
  dataIn_21/1 -> [dataIn_21]
  dataIn_23/1 -> [dataIn_23]
  dataIn_26/1 -> [dataIn_26]
  dataIn_30/1 -> [dataIn_30]
  dataIn_31/1 -> [dataIn_31]
  dataIn_32/1 -> [dataIn_32]
  dataIn_33/1 -> [dataIn_33]
  dataIn_37/1 -> [dataIn_37]
  dataIn_35/1 -> [dataIn_35]
  dataIn_34/1 -> [dataIn_34]
  dataIn_36/1 -> [dataIn_36]
  dataIn_38/1 -> [dataIn_38]
  dataIn_11/1 -> [dataIn_11]
  [dataIn_24] -> Comparator7/1
  [dataIn_13] -> Comparator3/2
  Comparator3/1 -> [result_13]
  [dataIn_24] -> Comparator4/1
  [dataIn_24] -> Comparator3/1
  [dataIn_24] -> Comparator5/1
  Comparator5/1 -> [result_15]
  [dataIn_14] -> Comparator4/2
  [dataIn_15] -> Comparator5/2
  Comparator4/1 -> [result_14]
  [dataIn_24] -> Comparator27/1
  [dataIn_24] -> Comparator28/1
  [dataIn_24] -> Comparator31/1
  [dataIn_32] -> Comparator31/2
  [dataIn_24] -> Comparator32/1
  [dataIn_33] -> Comparator32/2
  [dataIn_24] -> Comparator33/1
  Comparator32/1 -> [result_33]
  Comparator27/1 -> [result_30]
  Comparator28/1 -> [result_31]
  Comparator31/1 -> [result_32]
  [dataIn_30] -> Comparator27/2
  [dataIn_31] -> Comparator28/2
  [dataIn_35] -> Comparator34/2
  Comparator35/1 -> [result_36]
  Comparator34/1 -> [result_35]
  [dataIn_34] -> Comparator33/2
  [dataIn_24] -> Comparator35/1
  Comparator29/1 -> [result_37]
  [dataIn_24] -> Comparator30/1
  [dataIn_36] -> Comparator35/2
  Comparator30/1 -> [result_38]
  [dataIn_24] -> Comparator34/1
  [dataIn_24] -> Comparator29/1
  [dataIn_37] -> Comparator29/2
  [dataIn_38] -> Comparator30/2
  Comparator33/1 -> [result_34]
  [result_13] -> Logical Bit Operator3/4
  [result_17] -> Logical Bit Operator3/8
  [result_14] -> Logical Bit Operator3/5
  [result_15] -> Logical Bit Operator3/6
  [result_16] -> Logical Bit Operator3/7
  [result_18] -> Logical Bit Operator3/9
  [result_12] -> Logical Bit Operator3/3
  Constant/1 -> Comparator6/1
  [result_24] -> Logical Bit Operator1/1
  [result_27] -> Logical Bit Operator4/7
  Constant1/1 -> Comparator7/2
  Comparator6/1 -> Logical Bit Operator/1
  [dataIn_24] -> Comparator12/1
  [dataIn_25] -> Comparator19/2
  Comparator13/1 -> [result_21]
  Comparator19/1 -> [result_25]
  [dataIn_24] -> Comparator19/1
  [dataIn_20] -> Comparator12/2
  [dataIn_24] -> Comparator16/1
  [dataIn_24] -> Comparator14/1
  [dataIn_24] -> Comparator13/1
  Comparator16/1 -> [result_22]
  [dataIn_22] -> Comparator16/2
  Comparator14/1 -> [result_27]
  [dataIn_24] -> Comparator17/1
  [dataIn_23] -> Comparator17/2
  [dataIn_24] -> Comparator15/1
  [dataIn_27] -> Comparator14/2
  Comparator17/1 -> [result_23]
  [dataIn_28] -> Comparator15/2
  [dataIn_26] -> Comparator20/2
  Comparator12/1 -> [result_20]
  [dataIn_24] -> Comparator20/1
  Comparator15/1 -> [result_28]
  Comparator20/1 -> [result_26]
  [dataIn_21] -> Comparator13/2
  [isKeyPoint] -> is_KeyPoint/1
  dataIn_12/1 -> [dataIn_12]
  dataIn_13/1 -> [dataIn_13]
  Comparator/1 -> [result_10]
  Logical Bit Operator4/1 -> Logical Bit Operator5/2
  Logical Bit Operator3/1 -> To Workspace/1, Logical Bit Operator5/1
  Logical Bit Operator2/1 -> Logical Bit Operator5/3
  Logical Bit Operator5/1 -> [isMax]
  Logical Bit Operator/1 -> [result_24]
  Logical Bit Operator1/1 -> [isKeyPoint]
